simulink model "current_sensor"  (R2022b)
settings: Solver=FixedStepAuto  StartTime=0.0  StopTime=10.0  RelTol=1e-3
undefined symbols (not defined in the file or in its folder): current_filter_order, fl_current, fs_current, N, offset_current, var_current
settings Model: Creator=aceao  LastModifiedBy=ramuj

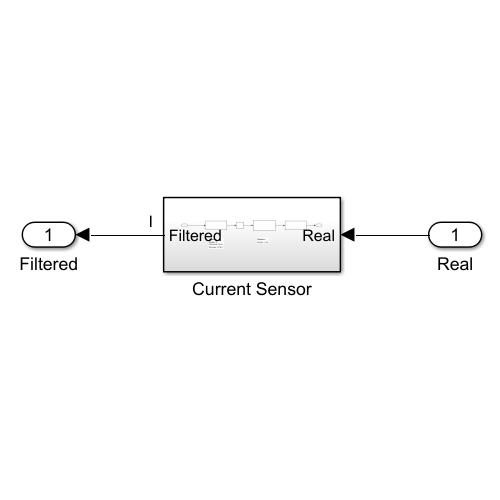
[thumbnail: Simulink's stored preview of the top-level diagram]
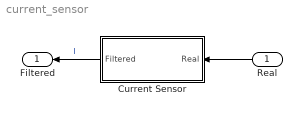
== system current_sensor ==
  Real : Inport
  Current Sensor : Subsystem
  Filtered : Outport
  wires:
  Real/1 -> Current Sensor/1(Real)
  Current Sensor/1(Filtered) -> Filtered/1  "I"

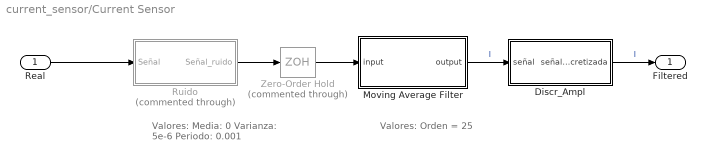
== system current_sensor/Current Sensor ==
  note: Valores:
      | Media: 0
      | Varianza: 5e-6
      | Periodo: 0.001
  note: Valores:
      | Orden = 25
  Real : Inport
  Discr_Ampl : Subsystem  mask{N=(2^N)-1, Min=-50, Max=50}
      mask prompts: N "Valores distintos (N)"; Min "Valor mínimo"; Max "Valor máximo"
      mask DialogControl DescGroupVar Prompt: Discretizacion_Amplitud
      mask DialogControl DescTextVar Prompt: Discretización en amplitud
  Moving Average Filter : Subsystem  mask{M=current_filter_order, fs=-1}
      mask prompts: M "Orden del filtro (M)"; fs "Frecuencia de muestreo (fs)"
  Ruido : Subsystem  Commented=through  mask{M=offset_current, V=var_current, T=1/fs_current}
      mask prompts: M "Media"; V "Varianza"; T "Periodo"
      mask DialogControl Ruido Prompt: Ruido
      mask DialogControl DescTextVar Prompt: Añade ruido gaussiano
  Zero-Order Hold : ZeroOrderHold  Commented=through  SampleTime=1/fl_current
  Filtered : Outport
  wires:
  Real/1 -> Ruido/1(Señal)
  Discr_Ampl/1(señal_discretizada) -> Filtered/1  "I"
  Moving Average Filter/1(output) -> Discr_Ampl/1(señal)  "I"
  Ruido/1(Señal_ruido) -> Zero-Order Hold/1
  Zero-Order Hold/1 -> Moving Average Filter/1(input)

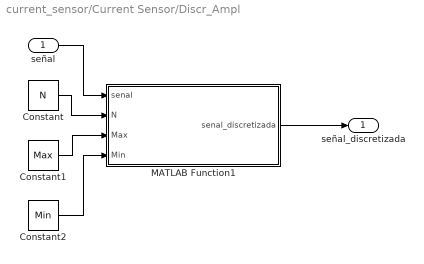
== system current_sensor/Current Sensor/Discr_Ampl ==
  señal : Inport
  Constant : Constant  Value=N
  Constant1 : Constant  Value=Max
  Constant2 : Constant  Value=Min
  MATLAB Function1 : MATLAB Function  TreatAsAtomicUnit=on
  señal_discretizada : Outport
  wires:
  MATLAB Function1/1(senal_discretizada) -> señal_discretizada/1
  señal/1 -> MATLAB Function1/1(senal)
  Constant1/1 -> MATLAB Function1/3(Max)
  Constant/1 -> MATLAB Function1/2(N)
  Constant2/1 -> MATLAB Function1/4(Min)

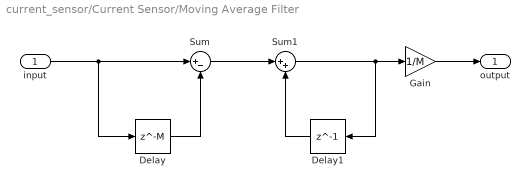
== system current_sensor/Current Sensor/Moving Average Filter ==
  input : Inport
  Delay : Delay  DelayLength=M  SampleTime=fs
  Delay1 : Delay  DelayLength=1  SampleTime=fs
  Gain : Gain  Gain=1/M
  Sum : Sum  Inputs=|+-
  Sum1 : Sum  Inputs=|++
  output : Outport
  wires:
  input/1 -> Delay/1, Sum/1
  Delay/1 -> Sum/2
  Sum/1 -> Sum1/1
  Sum1/1 -> Delay1/1, Gain/1
  Delay1/1 -> Sum1/2
  Gain/1 -> output/1

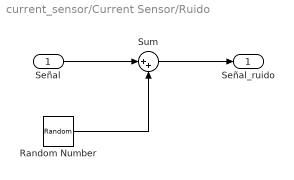
== system current_sensor/Current Sensor/Ruido ==
  Señal : Inport
  Random Number : RandomNumber  Mean=M  Variance=V  Seed=3  SampleTime=T
  Sum : Sum  Inputs=|++
  Señal_ruido : Outport
  wires:
  Random Number/1 -> Sum/2
  Señal/1 -> Sum/1
  Sum/1 -> Señal_ruido/1

== matlab function current_sensor/Current Sensor/Discr_Ampl/MATLAB Function1 ==
  data: senal input; senal_discretizada output; N input; Max input; Min input
function senal_discretizada  = fcn(senal,N,Max,Min)

if(senal>Max)
    senal_discretizada=Max;
    return
elseif(senal<Min)
    senal_discretizada=Min;
    return
end

valor_escalon=(Max-Min)/(N-1);
i=Min;
 while(i<Max)
    if(i+valor_escalon/2>senal)
        senal_discretizada=i;
        return
    end
    i=i+valor_escalon;
end

      senal_discretizada=Max;
end
